simulink model "genCmotorDiesel"  (R2017a)
settings: Solver=FixedStepDiscrete  StartTime=0.0  StopTime=1000  FixedStep=0.01  RelTol=1e-3  EnableMultiTasking=on
libraries: rtwdemowidgets x2
Description:
  | Customizing a Main Program for Your Target
  | 
  | This model shows the "Generate an example main program"
  | feature of Embedded Coder(R).
settings Model: ExtModeArmWhenConnect=off  ExtModeAutoUpdateStatusClock=off  Creator=The MathWorks, Inc.  LastModifiedBy=Administrador
settings DataIOCC: LimitDataPoints=on  SaveFormat=Array  SaveOutput=off  SaveTime=off  SignalLoggingName=sigsOut
settings OptimizationCC: DefaultParameterBehavior=Inlined  UseDivisionForNetSlopeComputation=on  InlineInvariantSignals=on  EnhancedBackFolding=on  PassReuseOutputArgsAs=Individual arguments  ExpressionDepthLimit=2147483647  StateBitsets=on  DataBitsets=on  EfficientFloat2IntCast=on
settings DebuggingCC: UnderspecifiedInitializationDetection=Classic  MergeDetectMultiDrivingBlocksExec=none  CheckExecutionContextPreStartOutputMsg=on  CheckExecutionContextRuntimeOutputMsg=on  ParameterTunabilityLossMsg=error  FcnCallInpInsideContextMsg=warning  UnconnectedInputMsg=none  UnconnectedOutputMsg=none  UnconnectedLineMsg=none  AllowSymbolicDim=off  StateNameClashWarn=warning  StrictBusMsg=ErrorOnBusTreatedAsVector  SFUnexpectedBacktrackingDiag=warning  SFNoUnconditionalDefaultTransitionDiag=warning  SFExecutionAtInitializationDiag=none
settings HardwareCC: ProdLargestAtomicFloat=None  ProdLongLongMode=on  ProdHWDeviceType=Specified  TargetBitPerPointer=64  TargetBitPerSizeT=64  TargetBitPerPtrDiffT=64  TargetLongLongMode=on  TargetIntDivRoundTo=Zero  TargetEndianess=LittleEndian  TargetWordSize=64  TargetHWDeviceType=MATLAB Host  ProdEqTarget=off
settings ModelReferenceCC: PropagateSignalLabelsOutOfModel=off
settings SFSimCC: MATLABDynamicMemAlloc=off
settings RTWCC: SystemTargetFile=ert.tlc  TLCOptions=-p0 -aWarnNonSaturatedBlocks=0  TemplateMakefile=ert_default_tmf  Description=Embedded Coder  GenerateReport=on  RTWVerbose=off  IncludeHyperlinkInReport=on  LaunchReport=on  GenerateTraceInfo=on  GenerateTraceReport=on  GenerateTraceReportSl=on  GenerateTraceReportSf=on  GenerateTraceReportEml=on
settings CodeAppCC: ForceParamTrailComments=on  IgnoreCustomStorageClasses=off  OperatorAnnotations=on  SimulinkDataObjDesc=on  SFDataObjDesc=on  MATLABFcnDesc=on  InsertBlockDesc=on  MATLABSourceComments=on
settings ERTTargetCC: GenerateSampleERTMain=on  MatFileLogging=on  InlinedParameterPlacement=NonHierarchical  ERTCustomFileTemplate=example_file_process.tlc
settings ConfigComp: CovMetricSettings=dw  CovHtmlReporting=on  CovSaveCumulativeToWorkspaceVar=on  CovSaveSingleToWorkspaceVar=on  CovExternalEMLEnable=off

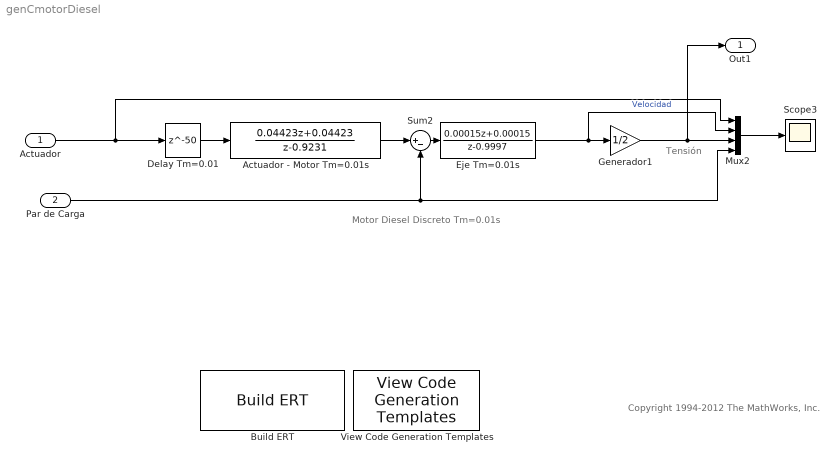
== system genCmotorDiesel ==
  note: Copyright 1994-2012 The MathWorks, Inc.
  note: Motor Diesel Discreto Tm=0.01s
  note: Tensión
  Actuador : Inport  OutDataTypeStr=double  PortDimensions=1  SampleTime=0.01
  Par de Carga : Inport  Port=2  OutDataTypeStr=double  PortDimensions=1  SampleTime=0.01
  " Generador1" : Gain  Gain=1/2
  Actuador - Motor Tm=0.01s : DiscreteTransferFcn  Numerator=[0.04423 0.04423]  Denominator=[1 -0.9231]  SampleTime=0.01
  Build ERT : rtwdemowidgets/Build ERT  attrib_overrides={'TargetOS'}
  Delay Tm=0.01 : Delay  DelayLength=50  SampleTime=0.01
  Eje Tm=0.01s : DiscreteTransferFcn  Numerator=[0.00015 0.00015]  Denominator=[1 -0.9997]  SampleTime=0.01
  Mux2 : Mux
  Scope3 : Scope
  Sum2 : Sum  Inputs=|+-
  View Code Generation Templates : rtwdemowidgets/View Code Generation Templates  SystemSampleTime=-1
  Out1 : Outport
  wires:
  Actuador - Motor Tm=0.01s/1 -> Sum2/1
  Delay Tm=0.01/1 -> Actuador - Motor Tm=0.01s/1
  Eje Tm=0.01s/1 -> Mux2/2, " Generador1"/1  "Velocidad"
  Mux2/1 -> Scope3/1
  Sum2/1 -> Eje Tm=0.01s/1
  " Generador1"/1 -> Out1/1, Mux2/3
  Par de Carga/1 -> Mux2/4, Sum2/2
  Actuador/1 -> Delay Tm=0.01/1, Mux2/1
